simulink model "TILC_AirRef_v2_longlat_n"  (R2017b)
settings: Solver=ode4  StartTime=0.0  StopTime=Tend  FixedStep=Ts  RelTol=1e-5  EnableMultiTasking=on
values from neighbouring files (symbols this model uses):
  A_rc_lat_O = [ 0  393.7200  -45.4165  393.7200         0         0 ... (first row only)    [F16_v3_longlat.m]
  A_rc_long_O = [0      0            -2.55e-09	1               0               0 ... (first row only)    [F16_v3_longlat.m]
  B_rc_lat_O = [ 0         0 ... (first row only)    [F16_v3_longlat.m]
  B_rc_long_O = [0              0 ... (first row only)    [F16_v3_longlat.m]
  C_rc_lat_O = [ 1	0   0	0	0	0 ... (first row only)    [F16_v3_longlat.m]
  C_rc_long_O = [1	0   0	0	0	0 ... (first row only)    [F16_v3_longlat.m]
  Cdr_ = 0.8    [hose_parameter4dock.mat]
  dtheta10 = [0 0 0 0 0 0 0 0 0 0]    [hose_parameter4dock.mat]
  dtheta20 = [0 0 0 0 0 0 0 0 0 0]    [hose_parameter4dock.mat]
  height = 3000    [hose_parameter4dock.mat]
  k_reel = 0.5    [hose_parameter4dock.mat]
  Kp_lat_O = [-2.4334   -1235.6   81.670    -1103.7   -11.020   -64.389 ... (first row only)    [F16_v3_longlat.m]
  Kp_long_O = [2.4349    0.2668   53.4474    3.0008  -63.2722    0.1787 ... (first row only)    [F16_v3_longlat.m]
  l0 = 1.44444444444    [hose_parameter4dock.mat]
  l1 = 2    [hose_parameter4dock.mat]
  l_density = 4.1    [hose_parameter4dock.mat]
  m0 = 5.92222222222    [hose_parameter4dock.mat]
  Mdr = 29.5    [hose_parameter4dock.mat]
  N = 10    [hose_parameter4dock.mat]
  Rdr = 0.305    [hose_parameter4dock.mat]
  Rl = 0.0336    [hose_parameter4dock.mat]
  T_reel_initial = 1610    [hose_parameter4dock.mat]
  theta10 = [0.459903280115 0.432776206681 0.412025416789 0.390288667864 0.365355881715 0.340009787283 0.310854701374 0.281345523746 0.248396428993 0.214590627751]    [hose_parameter4dock.mat]
  theta20 = [0 0 0 0 0 0 0 0 0 0]    [hose_parameter4dock.mat]
  vt0 = [120 0 0]    [hose_parameter4dock.mat]
undefined symbols (not defined in the file or in its folder): d_f_rc, F, MIL, p0_rc, STD
libraries: simulink x7, aerolibwind2 x2, aerolibatmos2 x1
settings Model: Creator=WhisPer  LastModifiedBy=Jinrui
settings DataIOCC: LimitDataPoints=on  SaveFormat=Array
settings OptimizationCC: LifeSpan=inf
settings DebuggingCC: UnderspecifiedInitializationDetection=Classic  MergeDetectMultiDrivingBlocksExec=none  SolverPrmCheckMsg=warning  AllowSymbolicDim=off  StateNameClashWarn=warning  SFUnexpectedBacktrackingDiag=warning  SFNoUnconditionalDefaultTransitionDiag=warning  SFExecutionAtInitializationDiag=none
settings HardwareCC: ProdBitPerPointer=32  ProdBitPerSizeT=32  ProdBitPerPtrDiffT=32  ProdLargestAtomicFloat=None  ProdIntDivRoundTo=Undefined  ProdEndianess=Unspecified  ProdWordSize=32  ProdHWDeviceType=32-bit Generic
settings ModelReferenceCC: PropagateSignalLabelsOutOfModel=off
settings CodeAppCC: StateflowObjectComments=on
settings GRTTargetCC: TargetLangStandard=C89/C90 (ANSI)  GeneratePreprocessorConditionals=Disable all
settings ConfigComp: CovMetricSettings=dw  CovHtmlReporting=on  CovSaveCumulativeToWorkspaceVar=on  CovSaveSingleToWorkspaceVar=on  CovExternalEMLEnable=off

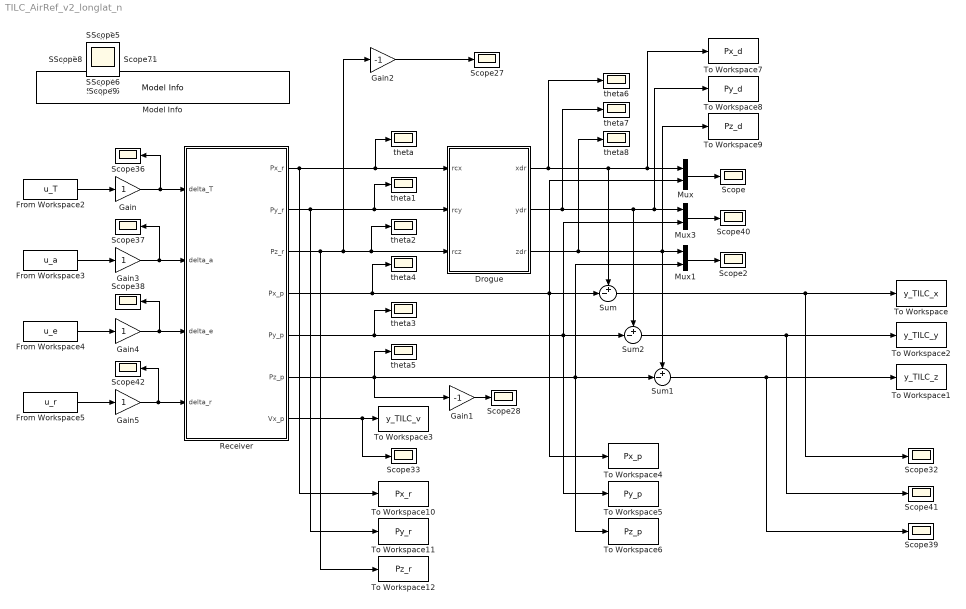
== system TILC_AirRef_v2_longlat_n ==
  Drogue : Subsystem
  From Workspace2 : FromWorkspace  VariableName=u_T  SampleTime=0
  From Workspace3 : FromWorkspace  VariableName=u_a  SampleTime=0
  From Workspace4 : FromWorkspace  VariableName=u_e  SampleTime=0
  From Workspace5 : FromWorkspace  VariableName=u_r  SampleTime=0
  Gain{,3..5} (4 alike) : Gain
  Gain1 : Gain  Gain=-1
  Gain2 : Gain  Gain=-1
  Model Info : simulink/Model-Wide Utilities/Model Info  Frame=on  DisplayStringWithTags=Run F16AirRef_Bowwave2Drogue_v2.slx first.  HorizontalTextAlignment=Center  LeftAlignmentValue=0.5
  Mux : Mux  Inputs=2
  Mux1 : Mux  Inputs=2
  Mux3 : Mux  Inputs=2
  Receiver : Subsystem
  Scope{,1..42} (43 alike) : Scope
  Sum : Sum  Inputs=+-|
  Sum1 : Sum  Inputs=+-|
  Sum2 : Sum  Inputs=+-|
  To Workspace : ToWorkspace  VariableName=y_TILC_x  SampleTime=-1
  To Workspace1 : ToWorkspace  VariableName=y_TILC_z  SampleTime=-1
  To Workspace10 : ToWorkspace  VariableName=Px_r  SampleTime=-1
  To Workspace11 : ToWorkspace  VariableName=Py_r  SampleTime=-1
  To Workspace12 : ToWorkspace  VariableName=Pz_r  SampleTime=-1
  To Workspace2 : ToWorkspace  VariableName=y_TILC_y  SampleTime=-1
  To Workspace3 : ToWorkspace  VariableName=y_TILC_v  SampleTime=-1
  To Workspace4 : ToWorkspace  VariableName=Px_p  SampleTime=-1
  To Workspace5 : ToWorkspace  VariableName=Py_p  SampleTime=-1
  To Workspace6 : ToWorkspace  VariableName=Pz_p  SampleTime=-1
  To Workspace7 : ToWorkspace  VariableName=Px_d  SampleTime=-1
  To Workspace8 : ToWorkspace  VariableName=Py_d  SampleTime=-1
  To Workspace9 : ToWorkspace  VariableName=Pz_d  SampleTime=-1
  theta{,1..8} (9 alike) : Scope
  wires:
  Drogue/1(xdr) -> theta6/1, To Workspace7/1, Mux/1, Sum/1
  Mux/1 -> Scope/1
  Mux1/1 -> Scope2/1
  Drogue/3(zdr) -> theta8/1, To Workspace9/1, Sum1/1, Mux1/1
  Receiver/3(Pz_r) -> To Workspace12/1, Gain2/1, theta2/1, Drogue/3(rcz)
  Receiver/4(Px_p) -> theta4/1, To Workspace4/1, Sum/2, Mux/2
  Receiver/6(Pz_p) -> Gain1/1, To Workspace6/1, Sum1/2, Mux1/2, theta5/1
  Gain2/1 -> Scope27/1
  Gain1/1 -> Scope28/1
  Sum/1 -> Scope32/1, To Workspace/1
  Sum1/1 -> Scope39/1, To Workspace1/1
  Receiver/1(Px_r) -> To Workspace10/1, theta/1, Drogue/1(rcx)
  Receiver/2(Py_r) -> To Workspace11/1, theta1/1, Drogue/2(rcy)
  Receiver/5(Py_p) -> theta3/1, To Workspace5/1, Mux3/2, Sum2/2
  Drogue/2(ydr) -> theta7/1, Sum2/1, To Workspace8/1, Mux3/1
  Sum2/1 -> Scope41/1, To Workspace2/1
  Mux3/1 -> Scope40/1
  Receiver/7(Vx_p) -> Scope33/1, To Workspace3/1
  From Workspace2/1 -> Gain/1
  From Workspace3/1 -> Gain3/1
  From Workspace4/1 -> Gain4/1
  From Workspace5/1 -> Gain5/1
  Gain/1 -> Receiver/1(delta_T), Scope36/1
  Gain4/1 -> Receiver/3(delta_e), Scope38/1
  Gain5/1 -> Receiver/4(delta_r), Scope42/1
  Gain3/1 -> Receiver/2(delta_a), Scope37/1

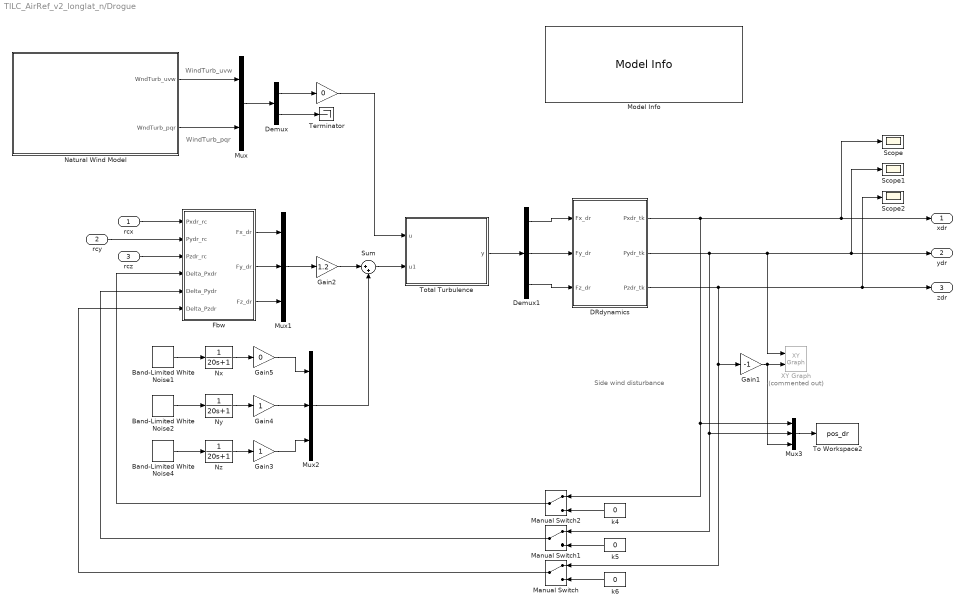
== system TILC_AirRef_v2_longlat_n/Drogue ==
  note: Side wind disturbance
  note: WindTurb_uvw
  note: WindTurb_pqr
  rcx : Inport
  rcy : Inport  Port=2
  rcz : Inport  Port=3
  " " : Gain  Gain=0
  Band-Limited White Noise1 : simulink/Sources/Band-Limited White Noise  Cov=[10]  Ts=0.1  seed=[23341]
  Band-Limited White Noise2 : simulink/Sources/Band-Limited White Noise  Cov=[10]  Ts=0.1  seed=[23341]
  Band-Limited White Noise4 : simulink/Sources/Band-Limited White Noise  Cov=[10]  Ts=0.1  seed=[23341]
  DRdynamics : Subsystem
  Demux : Demux  Outputs=2
  Demux1 : Demux  Outputs=3
  Fbw : Subsystem
  Gain1 : Gain  Gain=-1
  Gain2 : Gain  Gain=1.2
  Gain3 : Gain
  Gain4 : Gain
  Gain5 : Gain  Gain=0
  Manual Switch : ManualSwitch
  Manual Switch1 : ManualSwitch
  Manual Switch2 : ManualSwitch
  Model Info : simulink/Model-Wide Utilities/Model Info  Frame=on  DisplayStringWithTags=|  HorizontalTextAlignment=Center  LeftAlignmentValue=0.5
      | Set the tk-coordinate to 
      | the steady position of the drogue.
      | That means z towards the earth
      | Ppr_rc=[6.06 0.54 -0.86]
      | Pns_rc=[8.00 0.00  0.00]
      | Pfl_rc=[3.86 0.00 -0.86]
  Mux : Mux  Inputs=2
  Mux1 : Mux  Inputs=3
  Mux2 : Mux  Inputs=3
  Mux3 : Mux  Inputs=3
  "Natural Wind Model " : Subsystem
  Nx : TransferFcn  Denominator=[20 1]
  Ny : TransferFcn  Denominator=[20 1]
  Nz : TransferFcn  Denominator=[20 1]
  Scope : Scope
  Scope1 : Scope
  Scope2 : Scope
  Sum : Sum  Inputs=|++
  Terminator : Terminator
  To Workspace2 : ToWorkspace  VariableName=pos_dr  SampleTime=-1
  "Total Turbulence  " : MATLAB Function  TreatAsAtomicUnit=on
  XY Graph : simulink/Sinks/XY Graph  Commented=on  xmin=-1  xmax=1  ymin=-1  ymax=1  st=-1
  k4 : Constant  Value=0
  k5 : Constant  Value=0
  k6 : Constant  Value=0
  xdr : Outport
  ydr : Outport  Port=2
  zdr : Outport  Port=3
  wires:
  DRdynamics/1(Pxdr_tk) -> Mux3/1, Manual Switch2/1, Scope/1, xdr/1
  DRdynamics/2(Pydr_tk) -> Mux3/2, Manual Switch1/1, XY Graph/1, ydr/1, Scope1/1
  DRdynamics/3(Pzdr_tk) -> Scope2/1, zdr/1, Manual Switch/1, Gain1/1
  rcy/1 -> Fbw/2(Pydr_rc)
  rcz/1 -> Fbw/3(Pzdr_rc)
  Gain1/1 -> Mux3/3, XY Graph/2
  rcx/1 -> Fbw/1(Pxdr_rc)
  Manual Switch2/1 -> Fbw/4(Delta_Pxdr)
  Manual Switch1/1 -> Fbw/5(Delta_Pydr)
  Manual Switch/1 -> Fbw/6(Delta_Pzdr)
  k4/1 -> Manual Switch2/2
  k5/1 -> Manual Switch1/2
  k6/1 -> Manual Switch/2
  Mux3/1 -> To Workspace2/1
  "Natural Wind Model "/1(WndTurb_uvw) -> Mux/1
  "Natural Wind Model "/2(WndTurb_pqr) -> Mux/2
  Demux/1 -> " "/1
  Mux/1 -> Demux/1
  Demux/2 -> Terminator/1
  " "/1 -> "Total Turbulence  "/1(u)
  Fbw/2(Fy_dr) -> Mux1/2
  Fbw/1(Fx_dr) -> Mux1/1
  Fbw/3(Fz_dr) -> Mux1/3
  Mux1/1 -> Gain2/1
  "Total Turbulence  "/1(y) -> Demux1/1
  Demux1/2 -> DRdynamics/2(Fy_dr)
  Demux1/1 -> DRdynamics/1(Fx_dr)
  Demux1/3 -> DRdynamics/3(Fz_dr)
  Band-Limited White Noise4/1 -> Nz/1
  Band-Limited White Noise1/1 -> Nx/1
  Gain4/1 -> Mux2/2
  Nz/1 -> Gain3/1
  Band-Limited White Noise2/1 -> Ny/1
  Ny/1 -> Gain4/1
  Nx/1 -> Gain5/1
  Gain5/1 -> Mux2/1
  Gain3/1 -> Mux2/3
  Gain2/1 -> Sum/1
  Sum/1 -> "Total Turbulence  "/2(u1)
  Mux2/1 -> Sum/2

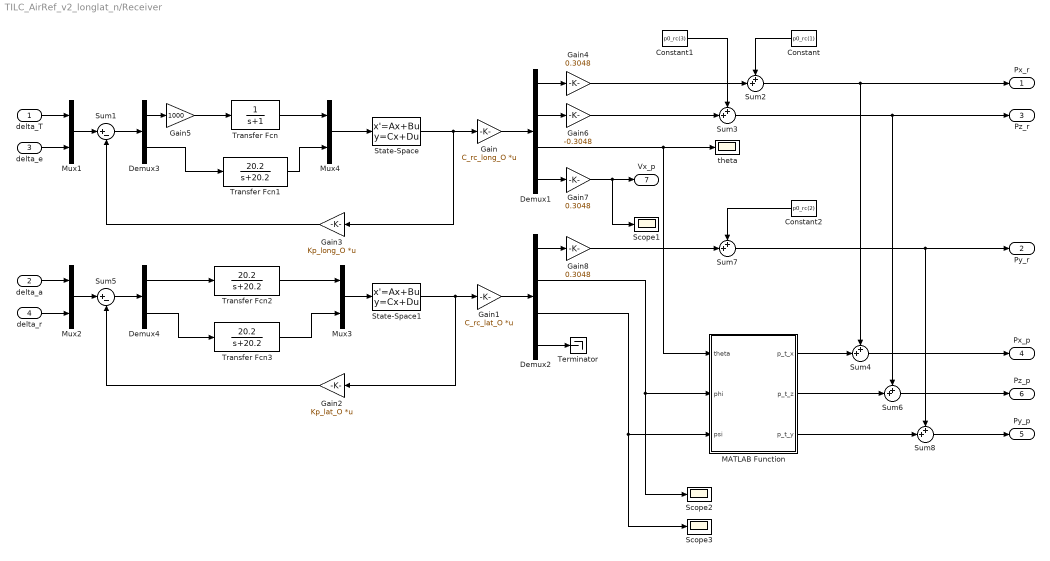
== system TILC_AirRef_v2_longlat_n/Receiver ==
  delta_T : Inport
  delta_a : Inport  Port=2
  delta_e : Inport  Port=3
  delta_r : Inport  Port=4
  Constant : Constant  Value=p0_rc(1)
  Constant1 : Constant  Value=p0_rc(3)
  Constant2 : Constant  Value=p0_rc(2)
  Demux1 : Demux
  Demux2 : Demux
  Demux3 : Demux  Outputs=2
  Demux4 : Demux  Outputs=2
  Gain : Gain  Gain=C_rc_long_O  Multiplication=Matrix(K*u) (u vector)
  Gain1 : Gain  Gain=C_rc_lat_O  Multiplication=Matrix(K*u) (u vector)
  Gain2 : Gain  Gain=Kp_lat_O  Multiplication=Matrix(K*u) (u vector)
  Gain3 : Gain  Gain=Kp_long_O  Multiplication=Matrix(K*u) (u vector)
  Gain4 : Gain  Gain=0.3048
  Gain5 : Gain  Gain=1000
  Gain6 : Gain  Gain=-0.3048
  Gain7 : Gain  Gain=0.3048
  Gain8 : Gain  Gain=0.3048
  MATLAB Function : MATLAB Function  TreatAsAtomicUnit=on
  Mux{1..4} (4 alike) : Mux  Inputs=2
  Scope1 : Scope
  Scope2 : Scope
  Scope3 : Scope
  State-Space : StateSpace  A=A_rc_long_O  B=0.6*B_rc_long_O  C=eye(6,6)  D=zeros(6,2)  InitialCondition=0
  State-Space1 : StateSpace  A=A_rc_lat_O  B=0.6*B_rc_lat_O  C=eye(6,6)  D=zeros(6,2)  InitialCondition=0
  Sum1 : Sum  Inputs=|+-
  Sum{2..4,6..8} (6 alike) : Sum  Inputs=++|
  Sum5 : Sum  Inputs=|+-
  Terminator : Terminator
  Transfer Fcn : TransferFcn  Denominator=[1 1]
  Transfer Fcn1 : TransferFcn  Numerator=[20.2]  Denominator=[1 20.2]
  Transfer Fcn2 : TransferFcn  Numerator=[20.2]  Denominator=[1 20.2]
  Transfer Fcn3 : TransferFcn  Numerator=[20.2]  Denominator=[1 20.2]
  theta : Scope
  Px_r : Outport
  Py_r : Outport  Port=2
  Pz_r : Outport  Port=3
  Px_p : Outport  Port=4
  Py_p : Outport  Port=5
  Pz_p : Outport  Port=6
  Vx_p : Outport  Port=7
  wires:
  Sum1/1 -> Demux3/1
  Demux3/1 -> Gain5/1
  Gain5/1 -> Transfer Fcn/1
  Mux4/1 -> State-Space/1
  State-Space/1 -> Gain3/1, Gain/1
  Gain3/1 -> Sum1/2
  Mux1/1 -> Sum1/1
  Gain/1 -> Demux1/1
  delta_T/1 -> Mux1/1
  delta_e/1 -> Mux1/2
  Demux1/3 -> MATLAB Function/1(theta), theta/1
  Sum2/1 -> Sum4/1, Px_r/1
  MATLAB Function/1(p_t_x) -> Sum4/2
  Sum4/1 -> Px_p/1
  Constant/1 -> Sum2/1
  Constant1/1 -> Sum3/1
  MATLAB Function/2(p_t_z) -> Sum6/2
  Sum3/1 -> Sum6/1, Pz_r/1
  Sum6/1 -> Pz_p/1
  Demux1/4 -> Gain7/1
  Demux1/1 -> Gain4/1
  Demux1/2 -> Gain6/1
  State-Space1/1 -> Gain2/1, Gain1/1
  Gain2/1 -> Sum5/2
  Mux2/1 -> Sum5/1
  delta_a/1 -> Mux2/1
  delta_r/1 -> Mux2/2
  Gain1/1 -> Demux2/1
  Demux2/4 -> Terminator/1
  Demux2/1 -> Gain8/1
  Sum7/1 -> Sum8/1, Py_r/1
  Constant2/1 -> Sum7/1
  Demux2/2 -> Scope2/1, MATLAB Function/2(phi)
  Demux2/3 -> Scope3/1, MATLAB Function/3(psi)
  MATLAB Function/3(p_t_y) -> Sum8/2
  Sum8/1 -> Py_p/1
  Gain4/1 -> Sum2/2
  Gain6/1 -> Sum3/2
  Gain7/1 -> Vx_p/1, Scope1/1
  Gain8/1 -> Sum7/2
  Transfer Fcn/1 -> Mux4/1
  Demux3/2 -> Transfer Fcn1/1
  Transfer Fcn1/1 -> Mux4/2
  Mux3/1 -> State-Space1/1
  Transfer Fcn2/1 -> Mux3/1
  Sum5/1 -> Demux4/1
  Demux4/1 -> Transfer Fcn2/1
  Demux4/2 -> Transfer Fcn3/1
  Transfer Fcn3/1 -> Mux3/2

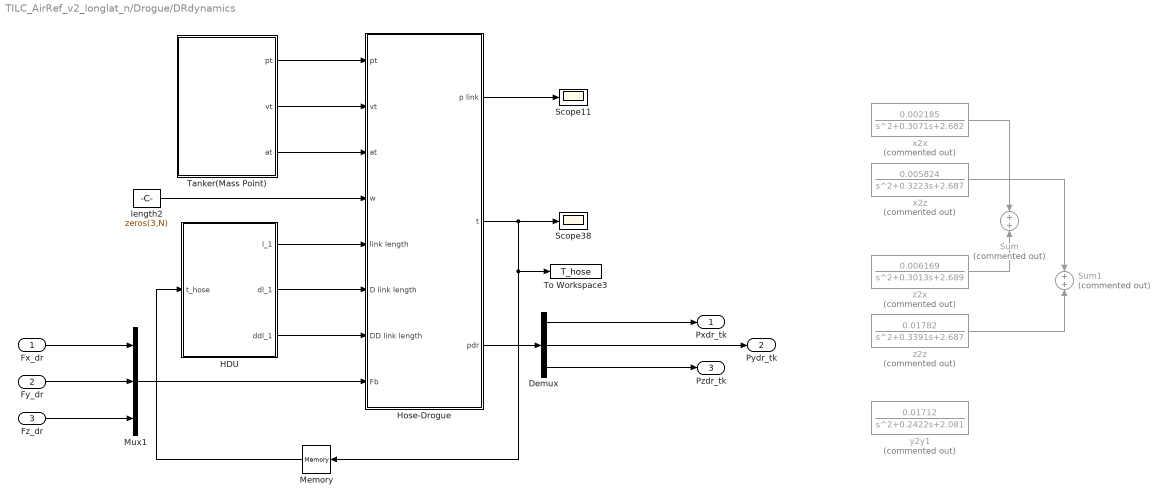
== system TILC_AirRef_v2_longlat_n/Drogue/DRdynamics ==
  Fx_dr : Inport
  Fy_dr : Inport  Port=2
  Fz_dr : Inport  Port=3
  Demux : Demux  Outputs=3
  HDU : Subsystem
  Hose-Drogue : Subsystem
  Memory : Memory  InitialCondition=T_reel_initial
  Mux1 : Mux  Inputs=3
  Scope11 : Scope
  Scope38 : Scope
  Sum : Sum  Commented=on  Inputs=+|+
  Sum1 : Sum  Commented=on  Inputs=+|+
  "Tanker(Mass Point) " : Subsystem
  To Workspace3 : ToWorkspace  VariableName=T_hose  SampleTime=-1
  length2 : Constant  Value=zeros(3,N)
  x2x : TransferFcn  Commented=on  Numerator=[0.002185]  Denominator=[1 0.3071 2.682]
  x2z : TransferFcn  Commented=on  Numerator=[0.005824]  Denominator=[1 0.3223 2.687]
  y2y1 : TransferFcn  Commented=on  Numerator=[0.01712]  Denominator=[1 0.2422 2.081]
  z2x : TransferFcn  Commented=on  Numerator=[0.006169]  Denominator=[1 0.3013 2.689]
  z2z : TransferFcn  Commented=on  Numerator=[0.01782]  Denominator=[1 0.3391 2.687]
  Pxdr_tk : Outport
  Pydr_tk : Outport  Port=2
  Pzdr_tk : Outport  Port=3
  wires:
  "Tanker(Mass Point) "/1(pt) -> Hose-Drogue/1(pt)
  "Tanker(Mass Point) "/2(vt) -> Hose-Drogue/2(vt)
  "Tanker(Mass Point) "/3(at) -> Hose-Drogue/3(at)
  length2/1 -> Hose-Drogue/4(w)
  Hose-Drogue/2(t) -> Scope38/1, Memory/1, To Workspace3/1
  Memory/1 -> HDU/1(t_hose)
  HDU/1(l_1) -> Hose-Drogue/5(link length)
  HDU/2(dl_1) -> Hose-Drogue/6(D link length)
  HDU/3(ddl_1) -> Hose-Drogue/7(DD link length)
  Hose-Drogue/1(p link) -> Scope11/1
  Mux1/1 -> Hose-Drogue/8(Fb)
  Fx_dr/1 -> Mux1/1
  Fy_dr/1 -> Mux1/2
  Fz_dr/1 -> Mux1/3
  Hose-Drogue/3(pdr) -> Demux/1
  Demux/1 -> Pxdr_tk/1
  Demux/2 -> Pydr_tk/1
  Demux/3 -> Pzdr_tk/1
  x2x/1 -> Sum/1
  z2x/1 -> Sum/2
  x2z/1 -> Sum1/1
  z2z/1 -> Sum1/2

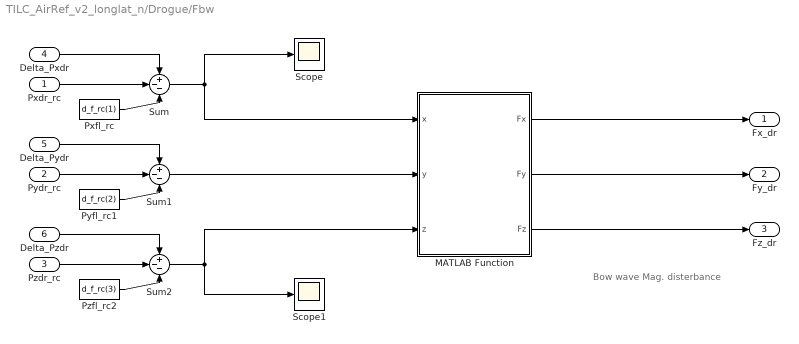
== system TILC_AirRef_v2_longlat_n/Drogue/Fbw ==
  note: Bow wave Mag. disterbance
  Pxdr_rc : Inport
  Pydr_rc : Inport  Port=2
  Pzdr_rc : Inport  Port=3
  Delta_Pxdr : Inport  Port=4
  Delta_Pydr : Inport  Port=5
  Delta_Pzdr : Inport  Port=6
  MATLAB Function : MATLAB Function  TreatAsAtomicUnit=on
  Pxfl_rc : Constant  Value=d_f_rc(1)
  Pyfl_rc1 : Constant  Value=d_f_rc(2)
  Pzfl_rc2 : Constant  Value=d_f_rc(3)
  Scope : Scope
  Scope1 : Scope
  Sum : Sum  Inputs=+--
  Sum1 : Sum  Inputs=+--
  Sum2 : Sum  Inputs=+--
  Fx_dr : Outport
  Fy_dr : Outport  Port=2
  Fz_dr : Outport  Port=3
  wires:
  Pxdr_rc/1 -> Sum/2
  Pxfl_rc/1 -> Sum/3
  Delta_Pxdr/1 -> Sum/1
  Pydr_rc/1 -> Sum1/2
  Delta_Pydr/1 -> Sum1/1
  Pyfl_rc1/1 -> Sum1/3
  Pzdr_rc/1 -> Sum2/2
  Pzfl_rc2/1 -> Sum2/3
  Delta_Pzdr/1 -> Sum2/1
  Sum/1 -> MATLAB Function/1(x), Scope/1
  Sum1/1 -> MATLAB Function/2(y)
  Sum2/1 -> MATLAB Function/3(z), Scope1/1
  MATLAB Function/2(Fy) -> Fy_dr/1
  MATLAB Function/3(Fz) -> Fz_dr/1
  MATLAB Function/1(Fx) -> Fx_dr/1

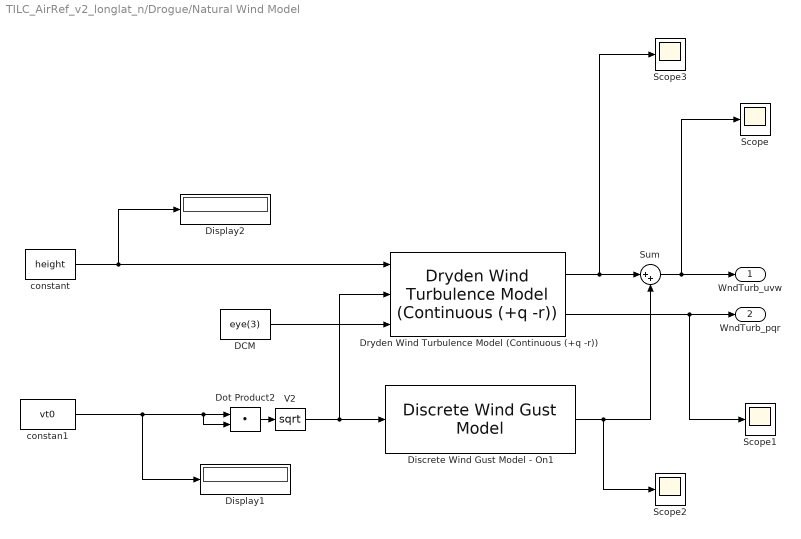
== system TILC_AirRef_v2_longlat_n/Drogue/Natural Wind Model  ==
  DCM : Constant  Value=eye(3)
  Discrete Wind Gust Model - On1 : aerolibwind2/Discrete Wind Gust Model  units=Metric (MKS)  Gx=on  Gy=on  Gz=on  t_0=600  d_m=[120 120 80]  v_m=[0 0 0]
      settings: SourceProductName=Aerospace Blockset
  Display1 : Display
  Display2 : Display
  Dot Product2 : DotProduct  SaturateOnIntegerOverflow=on  OutDataTypeStr=Inherit: Inherit via internal rule
  Dryden Wind Turbulence Model (Continuous (+q -r)) : aerolibwind2/Dryden Wind Turbulence Model  (Continuous (+q -r))  units=Metric (MKS)  spec=MIL-F-8785C  model=Continuous Dryden (+q -r)  W20=5  Wdeg=0  TurbProb=10^-1  L_high=5000  Wingspan=6  ts=0.1  Seed=1+fix(3650*rand(1,4))  T_on=on
      settings: SourceProductName=Aerospace Blockset
  Scope{,1..3} (4 alike) : Scope
  Sum : Sum  Inputs=|++  SaturateOnIntegerOverflow=on  InputSameDT=on  OutDataTypeStr=Inherit: Same as first input
  V2 : Math  Operator=sqrt  SaturateOnIntegerOverflow=on
  constan1 : Constant  Value=vt0
  constant : Constant  Value=height
  WndTurb_uvw : Outport
  WndTurb_pqr : Outport  Port=2
  wires:
  Sum/1 -> Scope/1, WndTurb_uvw/1
  Dryden Wind Turbulence Model (Continuous (+q -r))/2 -> Scope1/1, WndTurb_pqr/1
  DCM/1 -> Dryden Wind Turbulence Model (Continuous (+q -r))/3
  V2/1 -> Discrete Wind Gust Model - On1/1, Dryden Wind Turbulence Model (Continuous (+q -r))/2
  Dot Product2/1 -> V2/1
  constan1/1 -> Dot Product2/1, Dot Product2/2, Display1/1
  Discrete Wind Gust Model - On1/1 -> Scope2/1, Sum/2
  constant/1 -> Dryden Wind Turbulence Model (Continuous (+q -r))/1, Display2/1
  Dryden Wind Turbulence Model (Continuous (+q -r))/1 -> Scope3/1, Sum/1

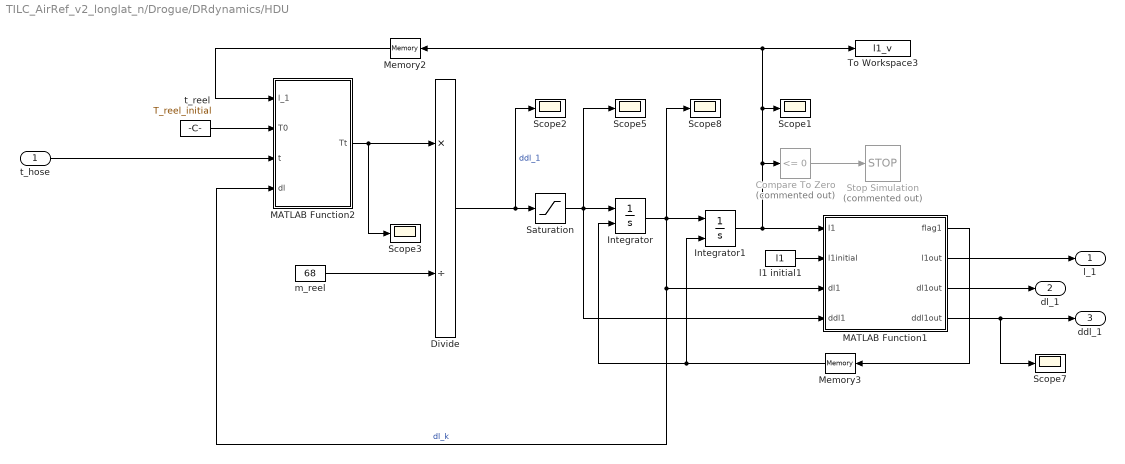
== system TILC_AirRef_v2_longlat_n/Drogue/DRdynamics/HDU ==
  t_hose : Inport
  Compare To Zero : simulink/Logic and Bit Operations/Compare To Zero  Commented=on  relop=<=  OutDataTypeStr=boolean
  Divide : Product  Inputs=*/
  Integrator : Integrator  ExternalReset=rising  UpperSaturationLimit=0.3  LowerSaturationLimit=-0.3
  Integrator1 : Integrator  ExternalReset=rising  InitialCondition=l1
  MATLAB Function1 : MATLAB Function  TreatAsAtomicUnit=on
  MATLAB Function2 : MATLAB Function  TreatAsAtomicUnit=on
  Memory2 : Memory  InitialCondition=l1
  Memory3 : Memory
  Saturation : Saturate  UpperLimit=3  LowerLimit=-3
  Scope{1..3,5,7..8} (6 alike) : Scope
  Stop Simulation : Stop  Commented=on
  To Workspace3 : ToWorkspace  VariableName=l1_v  SampleTime=-1
  l1 initial1 : Constant  Value=l1
  m_reel : Constant  Value=68
  t_reel : Constant  Value=T_reel_initial
  l_1 : Outport
  dl_1 : Outport  Port=2
  ddl_1 : Outport  Port=3
  wires:
  MATLAB Function2/1(Tt) -> Scope3/1, Divide/1
  m_reel/1 -> Divide/2
  Divide/1 -> Saturation/1, Scope2/1  "ddl_1"
  Integrator/1 -> Integrator1/1, MATLAB Function1/3(dl1), MATLAB Function2/4(dl), Scope8/1  "dl_k"
  Saturation/1 -> MATLAB Function1/4(ddl1), Integrator/1, Scope5/1
  t_reel/1 -> MATLAB Function2/2(T0)
  Compare To Zero/1 -> Stop Simulation/1
  l1 initial1/1 -> MATLAB Function1/2(l1initial)
  MATLAB Function1/4(ddl1out) -> Scope7/1, ddl_1/1
  MATLAB Function1/1(flag1) -> Memory3/1
  Memory2/1 -> MATLAB Function2/1(l_1)
  Memory3/1 -> Integrator/2, Integrator1/2
  Integrator1/1 -> MATLAB Function1/1(l1), Compare To Zero/1, To Workspace3/1, Memory2/1, Scope1/1
  MATLAB Function1/2(l1out) -> l_1/1
  MATLAB Function1/3(dl1out) -> dl_1/1
  t_hose/1 -> MATLAB Function2/3(t)

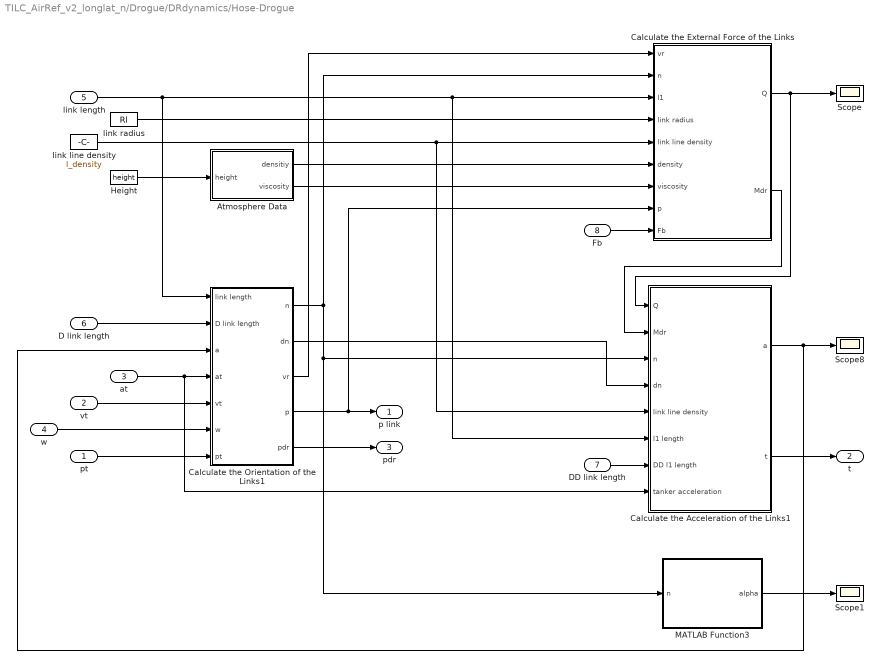
== system TILC_AirRef_v2_longlat_n/Drogue/DRdynamics/Hose-Drogue ==
  pt : Inport
  vt : Inport  Port=2
  at : Inport  Port=3
  w : Inport  Port=4
  link length : Inport  Port=5
  D link length : Inport  Port=6
  DD link length : Inport  Port=7
  Fb : Inport  Port=8
  Atmosphere Data : Subsystem
  Calculate the Acceleration of the Links1 : Subsystem
  Calculate the External Force of the Links : Subsystem
  Calculate the Orientation of the Links1 : Subsystem
  Height : Constant  Value=height
  MATLAB Function3 : MATLAB Function  TreatAsAtomicUnit=on
  Scope : Scope
  Scope1 : Scope
  Scope8 : Scope
  link line density : Constant  Value=l_density
  link radius : Constant  Value=Rl
  p link : Outport
  t : Outport  Port=2
  pdr : Outport  Port=3
  wires:
  Height/1 -> Atmosphere Data/1(height)
  Atmosphere Data/1(densitiy) -> Calculate the External Force of the Links/6(density)
  Atmosphere Data/2(viscosity) -> Calculate the External Force of the Links/7(viscosity)
  link radius/1 -> Calculate the External Force of the Links/4(link radius)
  link line density/1 -> Calculate the External Force of the Links/5(link line density), Calculate the Acceleration of the Links1/5(link line density)
  Calculate the External Force of the Links/1(Q) -> Scope/1, Calculate the Acceleration of the Links1/1(Q)
  Calculate the Orientation of the Links1/1(n) -> Calculate the External Force of the Links/2(n), MATLAB Function3/1(n), Calculate the Acceleration of the Links1/3(n)
  Calculate the Orientation of the Links1/2(dn) -> Calculate the Acceleration of the Links1/4(dn)
  Calculate the External Force of the Links/2(Mdr) -> Calculate the Acceleration of the Links1/2(Mdr)
  at/1 -> Calculate the Orientation of the Links1/4(at), Calculate the Acceleration of the Links1/8("tanker acceleration ")
  Calculate the Orientation of the Links1/3(vr) -> Calculate the External Force of the Links/1(vr)
  w/1 -> Calculate the Orientation of the Links1/6(w)
  Calculate the Acceleration of the Links1/1(a) -> Calculate the Orientation of the Links1/3(a), Scope8/1
  Calculate the Orientation of the Links1/4(p) -> Calculate the External Force of the Links/8(p), p link/1
  pt/1 -> Calculate the Orientation of the Links1/7(pt)
  vt/1 -> Calculate the Orientation of the Links1/5(vt)
  Calculate the Acceleration of the Links1/2(t) -> t/1
  link length/1 -> Calculate the Orientation of the Links1/1(link length), Calculate the External Force of the Links/3(l1), Calculate the Acceleration of the Links1/6(l1 length)
  D link length/1 -> Calculate the Orientation of the Links1/2(D link length)
  DD link length/1 -> Calculate the Acceleration of the Links1/7(DD l1 length)
  Fb/1 -> Calculate the External Force of the Links/9(Fb)
  MATLAB Function3/1(alpha) -> Scope1/1
  Calculate the Orientation of the Links1/5(pdr) -> pdr/1

== system TILC_AirRef_v2_longlat_n/Drogue/DRdynamics/Tanker(Mass Point)  ==
  Integrator : Integrator  InitialCondition=vt0
  Integrator1 : Integrator  InitialCondition=[0;0;0]
  tanker acceleration : Constant  Value=[0;0;0]
  pt : Outport
  vt : Outport  Port=2
  at : Outport  Port=3
  wires:
  tanker acceleration/1 -> at/1, Integrator/1
  Integrator/1 -> Integrator1/1, vt/1
  Integrator1/1 -> pt/1

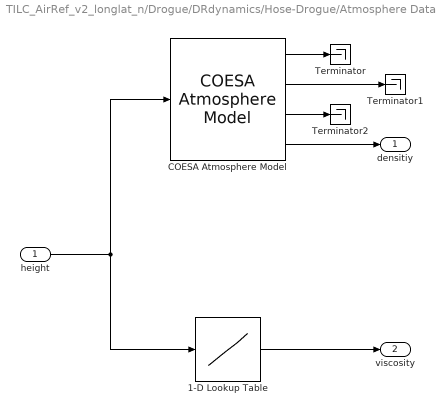
== system TILC_AirRef_v2_longlat_n/Drogue/DRdynamics/Hose-Drogue/Atmosphere Data ==
  height : Inport
  1-D Lookup Table : Lookup_n-D  NumberOfTableDimensions=1  BreakpointsForDimension1=[0,1000,2000,3000,4000,5000,6000,7000,8000,9000,10000]  Table=[1.789e-05,1.749e-05,1.717e-05,1.684e-05,1.652e-05,1.619e-05,1.586e-05,1.552e-05,1.517e-05,1.482e-05,1.447e-05]  RndMeth=Simplest  InputSameDT=on
  COESA Atmosphere Model : aerolibatmos2/COESA Atmosphere Model  units=Metric (MKS)  spec=MIL-STD-210C  model=Profile  profile_var=High temperature  profile_percent=1%  profile_alt=5 km (16404 ft)  envelope_var=High temperature  envelope_percent=1%  action=Warning
  Terminator : Terminator
  Terminator1 : Terminator
  Terminator2 : Terminator
  densitiy : Outport
  viscosity : Outport  Port=2
  wires:
  COESA Atmosphere Model/4 -> densitiy/1
  height/1 -> 1-D Lookup Table/1, COESA Atmosphere Model/1
  COESA Atmosphere Model/1 -> Terminator/1
  COESA Atmosphere Model/2 -> Terminator1/1
  COESA Atmosphere Model/3 -> Terminator2/1
  1-D Lookup Table/1 -> viscosity/1

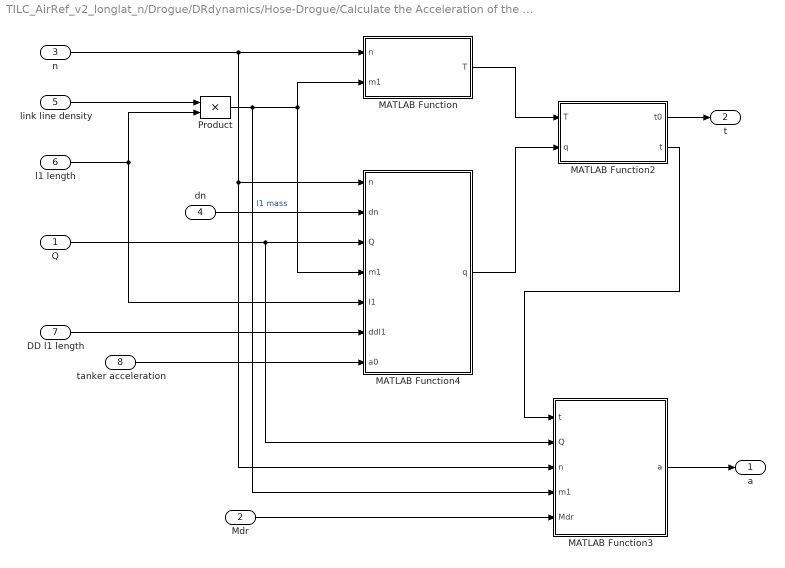
== system TILC_AirRef_v2_longlat_n/Drogue/DRdynamics/Hose-Drogue/Calculate the Acceleration of the Links1 ==
  Q : Inport
  Mdr : Inport  Port=2
  n : Inport  Port=3
  dn : Inport  Port=4
  link line density : Inport  Port=5
  l1 length : Inport  Port=6
  DD l1 length : Inport  Port=7
  "tanker acceleration " : Inport  Port=8
  MATLAB Function : MATLAB Function  TreatAsAtomicUnit=on
  MATLAB Function2 : MATLAB Function  TreatAsAtomicUnit=on
  MATLAB Function3 : MATLAB Function  TreatAsAtomicUnit=on
  MATLAB Function4 : MATLAB Function  TreatAsAtomicUnit=on
  Product : Product
  a : Outport
  t : Outport  Port=2
  wires:
  n/1 -> MATLAB Function4/1(n), MATLAB Function3/3(n), MATLAB Function/1(n)
  Product/1 -> MATLAB Function3/4(m1), MATLAB Function4/4(m1), MATLAB Function/2(m1)  "l1 mass"
  Q/1 -> MATLAB Function4/3(Q), MATLAB Function3/2(Q)
  DD l1 length/1 -> MATLAB Function4/6(ddl1)
  "tanker acceleration "/1 -> MATLAB Function4/7(a0)
  dn/1 -> MATLAB Function4/2(dn)
  l1 length/1 -> MATLAB Function4/5(l1), Product/2
  link line density/1 -> Product/1
  MATLAB Function/1(T) -> MATLAB Function2/1(T)
  MATLAB Function4/1(q) -> MATLAB Function2/2(q)
  MATLAB Function2/2(t) -> MATLAB Function3/1(t)
  Mdr/1 -> MATLAB Function3/5(Mdr)
  MATLAB Function3/1(a) -> a/1
  MATLAB Function2/1(t0) -> t/1

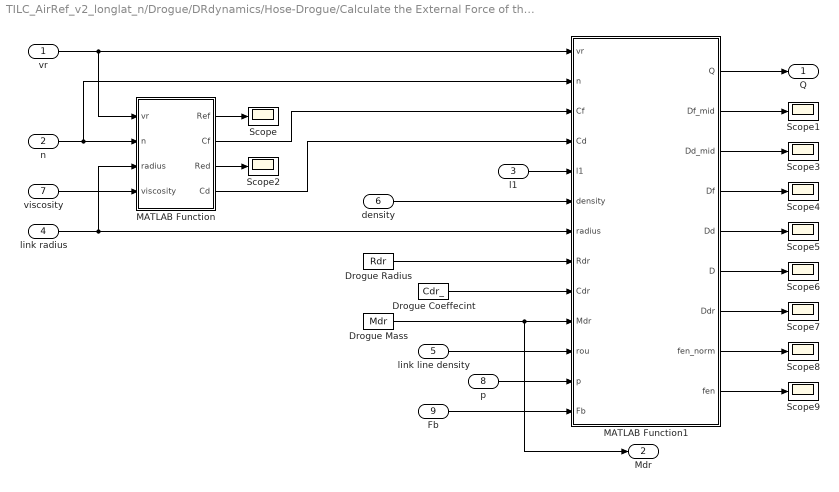
== system TILC_AirRef_v2_longlat_n/Drogue/DRdynamics/Hose-Drogue/Calculate the External Force of the Links ==
  vr : Inport
  n : Inport  Port=2
  l1 : Inport  Port=3
  link radius : Inport  Port=4
  link line density : Inport  Port=5
  density : Inport  Port=6
  viscosity : Inport  Port=7
  p : Inport  Port=8
  Fb : Inport  Port=9
  Drogue Coeffecint : Constant  Value=Cdr_
  Drogue Mass : Constant  Value=Mdr
  Drogue Radius : Constant  Value=Rdr
  MATLAB Function : MATLAB Function  TreatAsAtomicUnit=on
  MATLAB Function1 : MATLAB Function  TreatAsAtomicUnit=on
  Scope{,1..9} (10 alike) : Scope
  Q : Outport
  Mdr : Outport  Port=2
  wires:
  MATLAB Function/1(Ref) -> Scope/1
  MATLAB Function/3(Red) -> Scope2/1
  MATLAB Function1/1(Q) -> Q/1
  vr/1 -> MATLAB Function/1(vr), MATLAB Function1/1(vr)
  n/1 -> MATLAB Function1/2(n), MATLAB Function/2(n)
  link radius/1 -> MATLAB Function/3(radius), MATLAB Function1/7(radius)
  viscosity/1 -> MATLAB Function/4(viscosity)
  density/1 -> MATLAB Function1/6(density)
  Drogue Radius/1 -> MATLAB Function1/8(Rdr)
  Drogue Coeffecint/1 -> MATLAB Function1/9(Cdr)
  Drogue Mass/1 -> Mdr/1, MATLAB Function1/10(Mdr)
  link line density/1 -> MATLAB Function1/11(rou)
  MATLAB Function1/2(Df_mid) -> Scope1/1
  MATLAB Function1/3(Dd_mid) -> Scope3/1
  MATLAB Function1/4(Df) -> Scope4/1
  MATLAB Function1/5(Dd) -> Scope5/1
  MATLAB Function1/6(D) -> Scope6/1
  MATLAB Function1/7(Ddr) -> Scope7/1
  MATLAB Function/2(Cf) -> MATLAB Function1/3(Cf)
  MATLAB Function/4(Cd) -> MATLAB Function1/4(Cd)
  p/1 -> MATLAB Function1/12(p)
  l1/1 -> MATLAB Function1/5(l1)
  Fb/1 -> MATLAB Function1/13(Fb)
  MATLAB Function1/8(fen_norm) -> Scope8/1
  MATLAB Function1/9(fen) -> Scope9/1

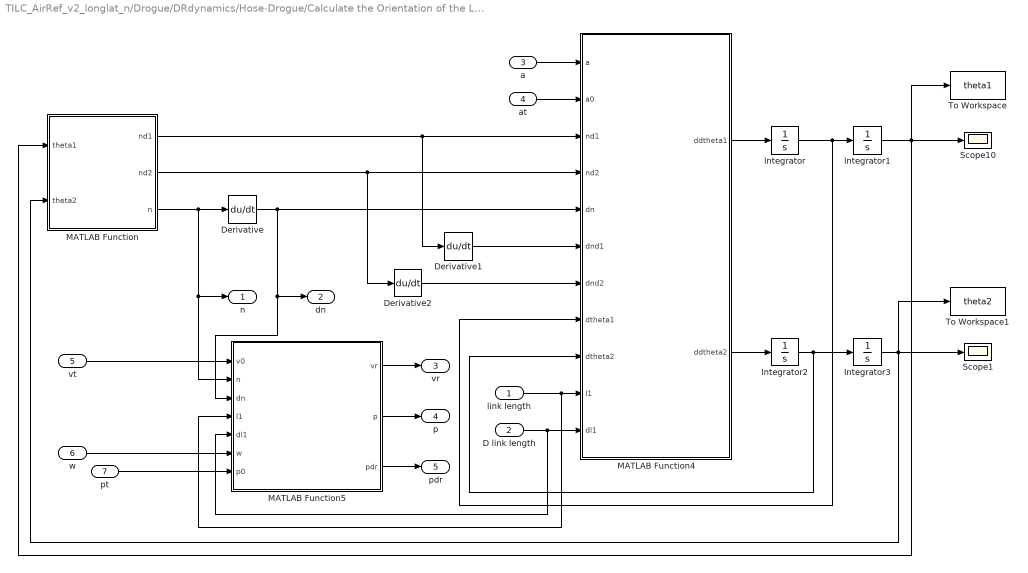
== system TILC_AirRef_v2_longlat_n/Drogue/DRdynamics/Hose-Drogue/Calculate the Orientation of the Links1 ==
  link length : Inport
  D link length : Inport  Port=2
  a : Inport  Port=3
  at : Inport  Port=4
  vt : Inport  Port=5
  w : Inport  Port=6
  pt : Inport  Port=7
  Derivative : Derivative
  Derivative1 : Derivative
  Derivative2 : Derivative
  Integrator : Integrator  InitialCondition=dtheta10
  Integrator1 : Integrator  InitialCondition=theta10
  Integrator2 : Integrator  InitialCondition=dtheta20
  Integrator3 : Integrator  InitialCondition=theta20
  MATLAB Function : MATLAB Function  TreatAsAtomicUnit=on
  MATLAB Function4 : MATLAB Function  TreatAsAtomicUnit=on
  MATLAB Function5 : MATLAB Function  TreatAsAtomicUnit=on
  Scope1 : Scope
  Scope10 : Scope
  To Workspace : ToWorkspace  VariableName=theta1  SampleTime=-1
      settings: Save2DSignal=2-D array (concatenate along first dimension)
  To Workspace1 : ToWorkspace  VariableName=theta2  SampleTime=-1
      settings: Save2DSignal=2-D array (concatenate along first dimension)
  n : Outport
  dn : Outport  Port=2
  vr : Outport  Port=3
  p : Outport  Port=4
  pdr : Outport  Port=5
  wires:
  Integrator1/1 -> To Workspace/1, MATLAB Function/1(theta1), Scope10/1
  Integrator3/1 -> To Workspace1/1, MATLAB Function/2(theta2), Scope1/1
  MATLAB Function/3(n) -> MATLAB Function5/2(n), n/1, Derivative/1
  Integrator/1 -> MATLAB Function4/8(dtheta1), Integrator1/1
  Integrator2/1 -> MATLAB Function4/9(dtheta2), Integrator3/1
  Derivative1/1 -> MATLAB Function4/6(dnd1)
  Derivative2/1 -> MATLAB Function4/7(dnd2)
  MATLAB Function4/1(ddtheta1) -> Integrator/1
  MATLAB Function4/2(ddtheta2) -> Integrator2/1
  link length/1 -> MATLAB Function4/10(l1), MATLAB Function5/4(l1)
  D link length/1 -> MATLAB Function5/5(dl1), MATLAB Function4/11(dl1)
  a/1 -> MATLAB Function4/1(a)
  at/1 -> MATLAB Function4/2(a0)
  vt/1 -> MATLAB Function5/1(v0)
  w/1 -> MATLAB Function5/6(w)
  MATLAB Function5/1(vr) -> vr/1
  pt/1 -> MATLAB Function5/7(p0)
  MATLAB Function5/2(p) -> p/1
  MATLAB Function/1(nd1) -> Derivative1/1, MATLAB Function4/3(nd1)
  MATLAB Function/2(nd2) -> Derivative2/1, MATLAB Function4/4(nd2)
  Derivative/1 -> MATLAB Function5/3(dn), dn/1, MATLAB Function4/5(dn)
  MATLAB Function5/3(pdr) -> pdr/1

== matlab function TILC_AirRef_v2_longlat_n/Receiver/MATLAB Function ==
  data: theta input; p_t_x output; phi input; psi input; d_pr_rc parameter; p_t_z output; p_t_y output
function [p_t_x,p_t_z,p_t_y] = fcn(theta,phi,psi,d_pr_rc)
%#codegen
R = [cos(theta)*cos(psi) sin(theta)*sin(phi)*cos(psi)-cos(phi)*sin(psi) sin(theta)*cos(phi)*cos(psi)+sin(phi)*sin(psi);
     cos(theta)*sin(psi) sin(theta)*sin(phi)*sin(psi)+cos(phi)*cos(psi) sin(theta)*cos(phi)*sin(psi)-sin(phi)*cos(psi);
     -sin(theta)         cos(theta)*sin(phi)                            cos(theta)*cos(phi)];
p = R*d_pr_rc;
p_t_x = p(1);
p_t_y = p(2);
p_t_z = p(3);

== matlab function TILC_AirRef_v2_longlat_n/Drogue/Fbw/MATLAB Function ==
  data: x input; Fx output; y input; z input; Fy output; Fz output
function [Fx,Fy,Fz] = F_rc2dr(x,y,z)

Cx1 = 91.6170;
Cx2 = 0.3220;
Cx3 = 3.8870;
Cx4 = 2.7359;
Cx5 = 2.4939;
Cx6 = 309.7709;
Cx7 = 0.3237;
Cx8 = 0.3851;
Cx9 = 1.1471;

Cy1 = 223.3210;
Cy2 = 0.2082;
Cy3 = 0.8102;
Cy4 = 0.6555;

Cz1 = 173.2021;
Cz2 = 0.2141;
Cz3 = 0.5697;
Cz4 = 0.7038;

% fz_o = -Cz1*(1-Cz2*xd_o)*exp(-yd_o^2/Cz3)*exp(zd_o/Cz4);
% 方向注意再查一下

if x > 5.6493
    Fx = 0;
elseif x > 3.0893
    Fx = Cx1*(1-Cx2*(x-Cx3)^2)*exp(-y^2/Cx4)*exp(z/Cx5);
else
    Fx = Cx1*(1-Cx2*(x-Cx3)^2)*exp(-y^2/Cx4)*exp(z/Cx5)...
       + Cx6*(1-Cx7*x)*exp(-y^2/Cx8)*exp(z/Cx9);
end

if x > 4.8031
    Fy = 0;
else
    Fy = Cy1*(1-Cy2*x)*(y*exp(-y^2/Cy3))*exp(z/Cy4);
end

if x > 4.6275
    Fz = 0;
else
    Fz = -Cz1*(1-Cz2*x)*exp(-y^2/Cz3)*exp(z/Cz4);
end

== matlab function TILC_AirRef_v2_longlat_n/Drogue/DRdynamics/Hose-Drogue/Calculate the External Force of the Links/MATLAB Function ==
  data: vr input; n input; Ref output; radius input; viscosity input; Cf output; Red output; Cd output; N parameter
function [Ref, Cf, Red, Cd] = C(vr,n,radius,viscosity, N)
% 计算雷诺数以及相应的摩擦系数Cf和压差系数Cd

% 单杆的速度、方向等用3*1的列向量表示
% vr = 连杆相对风速度 向量3*N
% n = 连杆的方向向量，想上为正 向量3*N
% viscosity  = 动粘度系数
% radius = 连杆半径

%——计算雷诺数———————————————————————————
cosa = zeros(1,N);
sina = zeros(1,N);
Ref = zeros(1,N);
Red = zeros(1,N);
for i = 1:N
    if norm(vr(:,i)) ~= 0
        cosa(i) = vr(:,i)'*n(:,i)/norm(vr(:,i));
        sina(i) = sqrt(1-cosa(i)^2);
        if sina(i) ~= 0
            Ref(i) = (pi*radius/viscosity)*norm(vr(:,i))/sina(i);
        else
            Ref(i) = 10^11;
        end
        Red(i) = norm(vr(:,i))*2*radius/viscosity;
    end
end

%——计算气动系数——————————————————————————
Cf = zeros(1,N);
Cd = zeros(1,N);
for i = 1:N
    %%%%Cf表%%%%%%%%%%%%%%%%%%%%%%%%
    if Ref(i)<=10^-2
        Cf(i) = 0;    %注意这里有改动
    elseif Ref(i)>10^-2 && Ref(i)<=10^4
        Cf(i) = 4.6409*Ref(i)^-0.6667;
    elseif Ref(i)>10^4 && Ref(i)<=10^10
        Cf(i) = 0.0464*Ref(i)^-0.1667;
    elseif Ref(i)>10^10
        Cf(i) = 0.001;
    end
    %%%%Cd表%%%%%%%%%%%%%%%%%%%%%%%%%
    if Red(i)<=10^-2
        Cd(i) = 0;   %注意这里有改动
    elseif Red(i)>10^-2 && Red(i)<=1
        Cd(i) = 10*Red(i)^-0.801;
    elseif Red(i)>1 && Red(i)<=180
        Cd(i) = 10*Red(i)^-0.4083;
    elseif Red(i)>180 && Red(i)<=4*10^5
        Cd(i) = 1.2;
    elseif Red(i)>4*10^5 && Red(i)<=4*10^6
        Cd(i) = 0.002128*Red(i)^0.3522;
    elseif Red(i)>4*10^6
        Cd(i) = 0.45;
    end
end

== matlab function TILC_AirRef_v2_longlat_n/Drogue/DRdynamics/Hose-Drogue/Calculate the External Force of the Links/MATLAB Function1 ==
  data: vr input; Q output; n input; Cf input; Cd input; l1 input; density input; radius input; Rdr input; Cdr input; Mdr input; rou input; p input; Fb input; Df_mid output; Dd_mid output; Df output; Dd output; D output; Ddr output; N parameter; l0 parameter; fen_norm output; fen output
function [Q, Df_mid, Dd_mid, Df, Dd, D, Ddr, fen_norm, fen] = ExternalForce(vr,n,Cf,Cd,l1,density,radius,Rdr,Cdr,Mdr,rou,p,Fb, N,l0)

% 计算每根连杆的合外力

% 单杆的速度、方向等用3*1的列向量表示
% l = 每根连杆的长度，注意这里要做成变长的 向量
% vr = 连杆相对风速度 向量3*N
% n = 连杆的方向向量，想上为正 向量3*N
% viscosity  = 大气动粘度系数
% density = 大气密度
% radius = 连杆半径
% r_dr = 锥套伞冠半径
% rou = 连杆的线密度

% Cdr = 锥套的阻力系数
% Rdr = 锥套伞冠半径
% Mdr = 锥套质量

%——求气动力————————————————————————————
Df_mid = zeros(1,N);
Dd_mid = zeros(1,N);
Df = zeros(3,N);
Dd = zeros(3,N);
D = zeros(3,N);
vn = zeros(3,N);
for i = 1:N
    if i == 1
        Df_mid(i) = density*pi*radius*l1*Cf(i)*(vr(:,i)'*n(:,i))^2;
    else
        Df_mid(i) = density*pi*radius*l0*Cf(i)*(vr(:,i)'*n(:,i))^2;
    end
    if vr(:,i)'*n(:,i)>0   % 这里可能有符号问题，万一之后还是出现杂乱的情况，要注意这里
        Df(:,i) = Df_mid(i)*n(:,i);
    else
        Df(:,i) = - Df_mid(i)*n(:,i);
    end
    % 当杆的方向迎着风的时候，摩擦阻力延杆反向
    % 当杆的方向顺着风的时候，摩擦阻力延杆正向
    
    vn(:,i) = vr(:,i)-(vr(:,i)'*n(:,i))*n(:,i); 
    if i == 1
        if norm(vn(:,i)) ~= 0
            Dd_mid(i) = density*radius*l1*Cd(i)*norm(vn(:,i))^2;
            Dd(:,i) = - Dd_mid(i)*vn(:,i)/norm(vn(:,i));
        else
            Dd(:,i) = [0;0;0];
        end
    else
        if norm(vn(:,i)) ~= 0
            Dd_mid(i) = density*radius*l0*Cd(i)*norm(vn(:,i))^2;
            Dd(:,i) = - Dd_mid(i)*vn(:,i)/norm(vn(:,i));
        else
            Dd(:,i) = [0;0;0];
        end
    end
    % 无论连杆与相对速度的角度关系如何，压差阻力总是顺着风的方向的
        
    D(:,i) = Df(:,i) + Dd(:,i);
end

if vr(:,N)'*vr(:,N) ~= 0
    Ddr = - 1/2*density*vr(:,N)'*vr(:,N)*(pi*Rdr^2)*(Cdr)* vr(:,N)/norm(vr(:,N));
else
    Ddr = [0;0;0];
end
%%%%%%%%%%%%%%%%%%%%%%%%%%%%%%%%%%%%%%%%%%%%%%%%%%%%%%%%%%%%%%%%

% %%%%计算恢复力%%%%%%%%%%%%%%%%%%%%%%
do = 1; % 连杆外径
di = 0.84; % 连杆内径
E = 589.67; % 弹性系数 数量级可能有问题
K = E*pi/8*(do^4 - di^4);
fen_norm = zeros(1,N);
fen = zeros(3,N);
for i = 2:N-1
    n0mid = (p(:,i-1) - p(:,i+1))/norm(p(:,i-1) - p(:,i+1));
    if abs(norm(n(:,i-1)'*n(:,i))-1) ~= 0;
        gama1 = n(:,i-1)'*n0mid;
        gama2 = n(:,i)'*n0mid;
        if norm(gama1) >= 1
            gama1 = gama1/abs(gama1);
        end
        if norm(gama2) >= 1
            gama2 = gama2/abs(gama2);
        end
            
        fen_norm(i) = K*(acos(gama1) + acos(gama2))/norm(p(:,i-1) - p(:,i+1))^2;
        fen(:,i) = fen_norm(i)*((n(:,i)'*n0mid*n0mid - n(:,i))*1e3)/norm((n(:,i)'*n0mid*n0mid - n(:,i))*1e3);
    end
end
%%%%%%%%%%%%%%%%%%%%%%%%%%%%%%%%%%%%%%

% %%%%计算合外力%%%%%%%%%%%%%%%%%%%%%%?
% Q = zeros(3,N);
% for i = 1:N-1
%     Q(:,i) = [0;0;m*g] + 1/2*(D(:,i)+D(:,i+1));
% end
% Q(:,N) = [0;0;(m+Mdr)*g] + 1/2*D(:,N) + Ddr;
Q = zeros(3,N);
Q(:,1) = [0;0;l1*rou*9.8] + 1/2*(D(:,1)+D(:,2)) + fen(:,1);
for i = 2:N-1
    Q(:,i) = [0;0;l0*rou*9.8] + 1/2*(D(:,i)+D(:,i+1)) + fen(:,i);
end
Q(:,N) = [0;0;(l0/2*rou + Mdr)*9.8] + 1/2*D(:,N) + Ddr + Fb;        %注意最后一个节点的质量
% 这里删掉了锥套的受力（Bow wave），后面再处理
% %%%%%%%%%%%%%%%%%%%%%%%%%%%%%%%%

== matlab function TILC_AirRef_v2_longlat_n/Drogue/DRdynamics/HDU/MATLAB Function1 ==
  data: l1 input; l1initial input; dl1 input; flag1 output size=1; l1out output; dl1out output; ddl1 input; ddl1out output
function [flag1,l1out,dl1out,ddl1out] = fcn(l1,l1initial,dl1,ddl1)

if (l1 > l1initial) || (l1 == l1initial && dl1 > 0)
    flag1 = 1;
    l1out = l1initial;
    dl1out = 0;
    ddl1out = 0;
else
    flag1 = 0;
    l1out = l1;
    dl1out = dl1;
    ddl1out = ddl1;
end

== matlab function TILC_AirRef_v2_longlat_n/Drogue/Total Turbulence   ==
  data: u input; u1 input; y output
function y = Dr_wnd2Frc(u,u1)
%#codegen

Ve=120;
rho = 0.98;
Q=0.5*rho*Ve^2;
S=0.38;
CD=0.81*0.8;

uu=u(1);
vv=u(2);
ww=u(3);

%beta = acos(sqrt(vv^2+ww^2)/abs(uu));
%theta = atan(ww/vv);

C_beta = 0.3979;

yx=rho*S*CD*Ve*uu;
yy=Q*S*C_beta*vv/Ve;
yz=Q*S*C_beta*ww/Ve;


y = [yx,yy,yz]';
y=u1+y;

== matlab function TILC_AirRef_v2_longlat_n/Drogue/DRdynamics/HDU/MATLAB Function2 ==
  data: l_1 input; T0 input; Tt output size=1; t input; dl input; l1 parameter; k_reel parameter
function Tt = fcn(l_1,T0,t,dl, l1,k_reel)
Treel = T0*(l_1/l1)^k_reel;
Tt = t - Treel - 500*dl;

== matlab function TILC_AirRef_v2_longlat_n/Drogue/DRdynamics/Hose-Drogue/MATLAB Function3 ==
  data: n input; alpha output; N parameter
function alpha = fcn(n, N)
% 计算两杆之间的弯折角度，用来粗略的验证恢复力的效果
alpha = zeros(1,N);
for i = 2:N
    mid = n(:,i-1)'*n(:,i);
    if abs(mid) > 1
        mid = mid/abs(mid);
    end
    alpha(i) = acos(mid)/pi*180;
end

== matlab function TILC_AirRef_v2_longlat_n/Drogue/DRdynamics/Hose-Drogue/Calculate the Acceleration of the Links1/MATLAB Function ==
  data: n input; m1 input; T output; m0 parameter; N parameter
function T = fcn(n,m1, m0,N)

% n = 连杆的方向向量，想上为正 向量3*N
% m = 连杆的质量 向量1*N

%%%%求张力t%%%%%%%%%%%%%%%%%%%%%%%%%%%%%%%%%%%%%%%%%%%%%%%%%%%%%%
T = zeros(N,N);

T(1,1) = 1;
T(1,2) = - n(:,1)'*n(:,2);
T(N,N-1) = -1/m0*n(:,N-1)'*n(:,N);
T(N,N) = 1/m0 + 1/m0;             %注意这里很重要！！

T(2,1) = -1/m1*n(:,1)'*n(:,2);
T(2,2) = 1/m1 + 1/m0;
T(2,3) = -1/m0*n(:,2)'*n(:,3);

for i = 3:N-1
    T(i,i-1) = -1/m0*n(:,i-1)'*n(:,i);
    T(i,i) = 1/m0 + 1/m0;
    T(i,i+1) = -1/m0*n(:,i)'*n(:,i+1);
end

== matlab function TILC_AirRef_v2_longlat_n/Drogue/DRdynamics/Hose-Drogue/Calculate the Orientation of the Links1/MATLAB Function ==
  data: nd1 output; nd2 output; theta1 input; n output; theta2 input; N parameter
function [nd1,nd2,n] = fcn(theta1,theta2, N)
% theta1,theta2 向量1*n
n = zeros(3,N);
nd1 = zeros(3,N);
nd2 = zeros(3,N);

for i = 1:N
    n(:,i) = [cos(theta1(i))*cos(theta2(i)); sin(theta2(i)); -sin(theta1(i))*cos(theta2(i))];
    nd1(:,i) = [-sin(theta1(i))*cos(theta2(i)); 0; -cos(theta1(i))*cos(theta2(i))];
    nd2(:,i) = [-cos(theta1(i))*sin(theta2(i)); cos(theta2(i)); sin(theta1(i))*sin(theta2(i))];
end

== matlab function TILC_AirRef_v2_longlat_n/Drogue/DRdynamics/Hose-Drogue/Calculate the Acceleration of the Links1/MATLAB Function2 ==
  data: t0 output size=1; T input; q input; t output
function [t0,t] = fcn(T,q)
t = T\q;
t0 = t(1);

== matlab function TILC_AirRef_v2_longlat_n/Drogue/DRdynamics/Hose-Drogue/Calculate the Acceleration of the Links1/MATLAB Function3 ==
  data: t input; Q input; n input; m1 input; Mdr input; a output; N parameter; m0 parameter
function a = fcn(t,Q,n,m1,Mdr, N,m0)
a = zeros(3,N);
a(:,1) = (t(1)*n(:,1) - t(2)*n(:,2) + Q(:,1))/m1;
for i = 2:N-1
    a(:,i) = (t(i)*n(:,i) - t(i+1)*n(:,i+1) + Q(:,i))/m0;
end
a(:,N) = (t(N)*n(:,N) + Q(:,N))/(m0/2 + Mdr);                %注意最后一个节点的质量！！

== matlab function TILC_AirRef_v2_longlat_n/Drogue/DRdynamics/Hose-Drogue/Calculate the Acceleration of the Links1/MATLAB Function4 ==
  data: n input; dn input; q output; Q input; m1 input; l1 input; ddl1 input; a0 input; N parameter; l0 parameter; m0 parameter
function q = fcn(n,dn,Q,m1,l1,ddl1,a0, N,l0,m0)

% n = 连杆的方向向量，想上为正 向量3*N
% Q = 连杆所受的合外力 向量3*N
% m = 连杆质量 向量1*N
% l = 连杆长度 向量1*N
% dl = 连杆长度的一阶导数 向量1*N
% ddl = 连杆长度的二阶导数 向量1*N
% a0 = 连接点的加速度 向量3*1

%%%%求张力t%%%%%%%%%%%%%%%%%%%%%%%%%%%%%%%%%%%%%%%%%%%%%%%%%%%%%%
q = zeros(N,1);
q(1,1) = m1*l1*dn(:,1)'*dn(:,1) - Q(:,1)'*n(:,1) + m1*a0'*n(:,1) - m1*ddl1;
q(2,1) = l0*dn(:,2)'*dn(:,2) + (1/m1*Q(:,1) - 1/m0*Q(:,2))'*n(:,2); % 可参考有关变长度连杆的《推导》
for i = 3:N
    q(i,1) = l0*dn(:,i)'*dn(:,i) + (1/m0*Q(:,i-1) - 1/m0*Q(:,i))'*n(:,i);
end

== matlab function TILC_AirRef_v2_longlat_n/Drogue/DRdynamics/Hose-Drogue/Calculate the Orientation of the Links1/MATLAB Function4 ==
  data: a input; a0 input; nd1 input; nd2 input; dn input; dnd1 input; dnd2 input; dtheta1 input; dtheta2 input; l1 input size=1; dl1 input; ddtheta1 output; ddtheta2 output; N parameter; l0 parameter
function [ddtheta1,ddtheta2] = fcn(a,a0,nd1,nd2,dn,dnd1,dnd2,dtheta1,dtheta2,l1,dl1, N, l0)
% theta1,theta2 向量N*1
% omiga,alpha是加油机坐标系的旋转角速度和叫加速度
% a是各节点的加速度
% a0为加油机加速度
% l,dl,ddl是连杆的长度及其一二阶导数

ddtheta1 = zeros(1,N);
ddtheta2 = zeros(1,N);

ddtheta1(1) = nd1(:,1)'*(-(a(:,1)-a0)-2*dl1*dn(:,1)-...
              l1*(dnd1(:,1)*dtheta1(1)+dnd2(:,1)*dtheta2(1)))...
              /(l1*norm(nd1(:,1)));
ddtheta2(1) = nd2(:,1)'*(-(a(:,1)-a0)-2*dl1*dn(:,1)-...
              l1*(dnd1(:,1)*dtheta1(1)+dnd2(:,1)*dtheta2(1)))...
              /(l1*norm(nd2(:,1)));
for i = 2:N
    ddtheta1(i) = nd1(:,i)'*(-(a(:,i)-a(:,i-1))-...
                  l0*(dnd1(:,i)*dtheta1(i)+dnd2(:,i)*dtheta2(i)))...
                  /(l0*norm(nd1(:,i)));
    ddtheta2(i) = nd2(:,i)'*(-(a(:,i)-a(:,i-1))-...
                  l0*(dnd1(:,i)*dtheta1(i)+dnd2(:,i)*dtheta2(i)))...
                  /(l0*norm(nd2(:,i)));
end

== matlab function TILC_AirRef_v2_longlat_n/Drogue/DRdynamics/Hose-Drogue/Calculate the Orientation of the Links1/MATLAB Function5 ==
  data: v0 input; n input; dn input; l1 input; dl1 input; w input; vr output; p0 input; p output; N parameter; l0 parameter; pdr output
function [vr,p,pdr] = fcn(v0,n,dn,l1,dl1,w,p0, N, l0)

% v0为加油机速度
% l,dl是连杆的长度及其一阶导数
% wt为合成风在每个节点的风速
% p0为预留，在计算相对地面的位置时用到

vr = zeros(3,N);
vr(:,1) = v0 - dl1*n(:,1) - l1*dn(:,1) ;
for i = 2:N
    vr(:,i) = vr(:,i-1) - l0*dn(:,i);
end
vr = vr - w;

p = zeros(3,N);
p(:,1) = [0;0;0] - l1*n(:,1);
for i = 2:N
    p(:,i) = p(:,i-1) - l0*n(:,i);
end
pdr = p(:,N) + [-0.3;0;0];
